simulink model "Glider_Sim_2015b"  (R2020a)
settings: Solver=ode45  StartTime=0.0  StopTime=10  MaxStep=0.1  RelTol=1e-3  EnableMultiTasking=on
InitFcn:
  | close all
  | AC=1; %Define Aircraft Case
  | SC_DynEqns; %Get the Stability Parameters
  | %[u alpha q theta beta p r phi]
  | XIC=[10. 6*pi/180. 0. 6*pi/180. 0*pi/180. 0. 0. 0*pi/180.]'; %Initial small perturbations
  | PsiIC=0.; %Initial Heading, radians
  | % clear the plot function to create new plots
  | % if you close the figure window, clear the function
  | % comment out the line below to overlay plots
  | clear PlotGlider
StartFcn:
  | tic
StopFcn:
  | toctime=toc;
  | xyz=xyz_E+[0 0 5000];
  | Score=0.3*(0.5*ceil(2*xyz(1))+4*abs(ceil(xyz(3))))+3*(abs(xyz(2))<=10);
  | fprintf('X-Dist = %5.1f    Score = %4.1f    Time= %3.1f sec\n',xyz(1),Score,tout(end))
  | str=(['X-Dist = ' num2str(xyz(1)) '    Score = ' num2str(Score)]);
values from neighbouring files (symbols this model uses):
  A = [Along zeros(4,4);zeros(4,4) Ald]    [SC_DynEqns.m]
  Alt = 5006    [AC_Data3.m]
  fps2kt = 0.5924838013    [AC_Data3.m]
  r2d = 180/pi    (= 57.2957795131)    [AC_Data3.m]
  tht = -0.086588    [AC_Data3.m]
  X0 = [U1 atrm 0 tht 0 0 0 0]'    [AC_Data3.m]
undefined symbols (not defined in the file or in its folder): PlotGlider
libraries: simulink x2
settings Model: Creator=bordignk  LastModifiedBy=Edward Han
settings DataIOCC: SaveFormat=Array  SignalLoggingSaveFormat=ModelDataLogs  ReturnWorkspaceOutputs=off
settings OptimizationCC: ExpressionDepthLimit=2147483647  InitFltsAndDblsToZero=on  LifeSpan=inf
settings DebuggingCC: UnderspecifiedInitializationDetection=Classic  MergeDetectMultiDrivingBlocksExec=none  FcnCallInpInsideContextMsg=warning  UnconnectedInputMsg=none  UnconnectedOutputMsg=none  AllowSymbolicDim=off  StateNameClashWarn=warning  SFUnexpectedBacktrackingDiag=warning  SFNoUnconditionalDefaultTransitionDiag=warning  SFExecutionAtInitializationDiag=none  ArithmeticOperatorsInVariantConditions=warning
settings HardwareCC: ProdBitPerPointer=32  ProdBitPerSizeT=32  ProdBitPerPtrDiffT=32  ProdLargestAtomicFloat=None  ProdIntDivRoundTo=Undefined  ProdEndianess=Unspecified  ProdWordSize=32  ProdHWDeviceType=32-bit Generic
settings ModelReferenceCC: PropagateSignalLabelsOutOfModel=off
settings SFSimCC: SimUseLocalCustomCode=off  SimParseCustomCode=off  CustomCodeUndefinedFunction=UseInterfaceOnly
settings RTWCC: RTWUseLocalCustomCode=off
settings CodeAppCC: StateflowObjectComments=on
settings GRTTargetCC: TargetLangStandard=C89/C90 (ANSI)  CombineOutputUpdateFcns=off  GRTInterface=on
settings ConfigComp: CovMetricSettings=dw  CovHtmlReporting=on  CovSaveCumulativeToWorkspaceVar=on  CovSaveSingleToWorkspaceVar=on  CovExternalEMLEnable=off  CovSFcnEnable=off

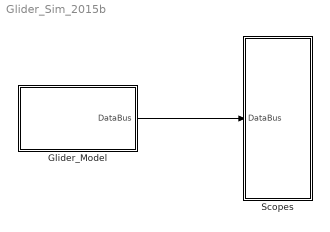
== system Glider_Sim_2015b ==
  Glider_Model : Subsystem
  Scopes : Subsystem
  wires:
  Glider_Model/1(DataBus) -> Scopes/1(DataBus)

== system Glider_Sim_2015b/Glider_Model ==
  Gain2 : Gain  Gain=A  Multiplication=Matrix(K*u)
  Integrator : Integrator  InitialCondition=XIC
  Make_Data : Subsystem
  DataBus : Outport  VectorParamsAs1DForOutWhenUnconnected=off
  wires:
  Gain2/1 -> Integrator/1, Make_Data/1(xdt)  "xdt"
  Make_Data/1(DataBus) -> DataBus/1
  Integrator/1 -> Make_Data/2(x)  "x"
  Make_Data/2(x_out) -> Gain2/1

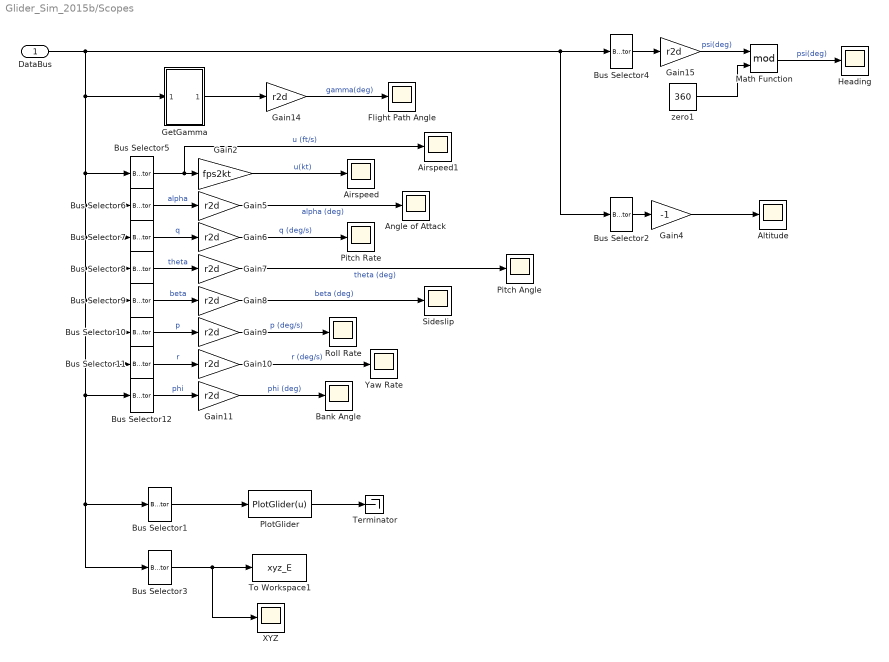
== system Glider_Sim_2015b/Scopes ==
  DataBus : Inport
  Airspeed : Scope
  Airspeed1 : Scope
  Altitude : Scope
  Angle of Attack : Scope
  Bank Angle : Scope
  Bus Selector1 : BusSelector  OutputSignals=Xe_ft,ye_ft,ze_ft,phi_rad,theta_rad,psi_rad  OutputAsBus=on
  Bus Selector10 : BusSelector  OutputSignals=p_rps  OutputAsBus=on
  Bus Selector11 : BusSelector  OutputSignals=r_rps  OutputAsBus=on
  Bus Selector12 : BusSelector  OutputSignals=phi_rad  OutputAsBus=on
  Bus Selector2 : BusSelector  OutputSignals=ze_ft  OutputAsBus=on
  Bus Selector3 : BusSelector  OutputSignals=Xe_ft,ye_ft,ze_ft  OutputAsBus=on
  Bus Selector4 : BusSelector  OutputSignals=psi_rad  OutputAsBus=on
  Bus Selector5 : BusSelector  OutputSignals=v_fps  OutputAsBus=on
  Bus Selector6 : BusSelector  OutputSignals=alpha_rad  OutputAsBus=on
  Bus Selector7 : BusSelector  OutputSignals=q_rps  OutputAsBus=on
  Bus Selector8 : BusSelector  OutputSignals=theta_rad  OutputAsBus=on
  Bus Selector9 : BusSelector  OutputSignals=beta_rad  OutputAsBus=on
  Flight Path Angle : Scope
  Gain{5..11,14..15} (9 alike) : Gain  Gain=r2d
  Gain2 : Gain  Gain=fps2kt
  Gain4 : Gain  Gain=-1
  GetGamma : Subsystem
  Heading : Scope
  Math Function : Math  Operator=mod  SignedPower=on  SaturateOnIntegerOverflow=on
  Pitch Angle : Scope
  Pitch Rate : Scope
  PlotGlider : MATLABFcn  MATLABFcn=PlotGlider(u)
  Roll Rate : Scope
  Sideslip : Scope
  Terminator : Terminator
  To Workspace1 : ToWorkspace  VariableName=xyz_E  SampleTime=-1
      settings: MaxDataPoints=1
  XYZ : Scope
  Yaw Rate : Scope
  zero1 : Constant  Value=360
  wires:
  DataBus/1 -> Bus Selector5/1, Bus Selector6/1, Bus Selector7/1, Bus Selector8/1, Bus Selector9/1, Bus Selector10/1, Bus Selector11/1, Bus Selector12/1, Bus Selector1/1, Bus Selector3/1, GetGamma/1(In1), Bus Selector4/1, Bus Selector2/1
  Math Function/1 -> Heading/1  "psi(deg)"
  Bus Selector2/1 -> Gain4/1
  Gain4/1 -> Altitude/1
  Bus Selector4/1 -> Gain15/1
  Bus Selector5/1 -> Airspeed1/1, Gain2/1  "u (ft/s)"
  Bus Selector6/1 -> Gain5/1  "alpha"
  Bus Selector7/1 -> Gain6/1  "q"
  Bus Selector8/1 -> Gain7/1  "theta"
  Bus Selector9/1 -> Gain8/1  "beta"
  Bus Selector10/1 -> Gain9/1  "p"
  Bus Selector11/1 -> Gain10/1  "r"
  Bus Selector12/1 -> Gain11/1  "phi"
  Gain5/1 -> Angle of Attack/1  "alpha (deg)"
  Gain6/1 -> Pitch Rate/1  "q (deg/s)"
  Gain7/1 -> Pitch Angle/1  "theta (deg)"
  Gain8/1 -> Sideslip/1  "beta (deg)"
  Gain9/1 -> Roll Rate/1  "p (deg/s)"
  Gain10/1 -> Yaw Rate/1  "r (deg/s)"
  Gain11/1 -> Bank Angle/1  "phi (deg)"
  Gain2/1 -> Airspeed/1  "u(kt)"
  Gain15/1 -> Math Function/1  "psi(deg)"
  zero1/1 -> Math Function/2
  Gain14/1 -> Flight Path Angle/1  "gamma(deg)"
  Bus Selector1/1 -> PlotGlider/1
  PlotGlider/1 -> Terminator/1
  GetGamma/1(Out1) -> Gain14/1
  Bus Selector3/1 -> XYZ/1, To Workspace1/1

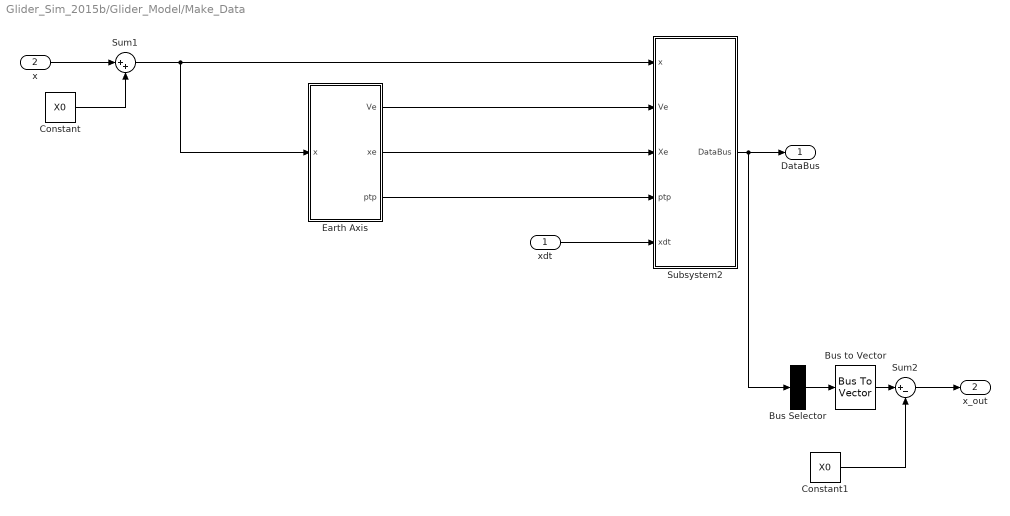
== system Glider_Sim_2015b/Glider_Model/Make_Data ==
  xdt : Inport  PortDimensions=[8 1]
  x : Inport  Port=2  PortDimensions=[8 1]
  Bus Selector : BusSelector  OutputSignals=v_fps,alpha_rad,q_rps,theta_rad,beta_rad,p_rps,r_rps,phi_rad  OutputAsBus=on
  Bus to Vector : BusToVector
  Constant : Constant  Value=X0
  Constant1 : Constant  Value=X0
  Earth Axis : Subsystem
  Subsystem2 : Subsystem
  Sum1 : Sum  Inputs=|++
  Sum2 : Sum  Inputs=|+-
  DataBus : Outport  VectorParamsAs1DForOutWhenUnconnected=off
  x_out : Outport  Port=2  VectorParamsAs1DForOutWhenUnconnected=off
  wires:
  x/1 -> Sum1/1
  Constant/1 -> Sum1/2
  Sum1/1 -> Subsystem2/1(x), Earth Axis/1(x)
  Earth Axis/2(xe) -> Subsystem2/3(Xe)
  xdt/1 -> Subsystem2/5(xdt)
  Subsystem2/1(DataBus) -> Bus Selector/1, DataBus/1
  Earth Axis/1(Ve) -> Subsystem2/2(Ve)
  Earth Axis/3(ptp) -> Subsystem2/4(ptp)
  Bus Selector/1 -> Bus to Vector/1
  Bus to Vector/1 -> Sum2/1
  Constant1/1 -> Sum2/2
  Sum2/1 -> x_out/1

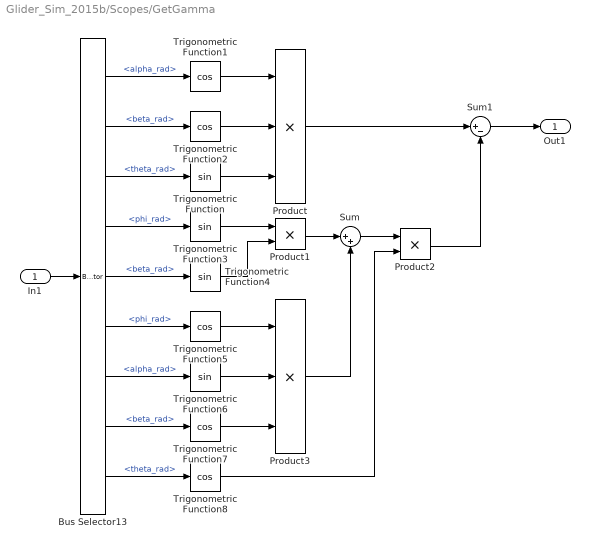
== system Glider_Sim_2015b/Scopes/GetGamma ==
  In1 : Inport
  Bus Selector13 : BusSelector  OutputSignals=alpha_rad,beta_rad,theta_rad,phi_rad,beta_rad,phi_rad,alpha_rad,beta_rad,theta_rad
  Product : Product  Inputs=3
  Product1 : Product
  Product2 : Product
  Product3 : Product  Inputs=3
  Sum : Sum  Inputs=|++
  Sum1 : Sum  Inputs=|+-
  Trigonometric Function{,3..4,6} (4 alike) : Trigonometry
  Trigonometric Function{1..2,5,7..8} (5 alike) : Trigonometry  Operator=cos
  Out1 : Outport  VectorParamsAs1DForOutWhenUnconnected=off
  wires:
  Sum1/1 -> Out1/1
  In1/1 -> Bus Selector13/1
  Bus Selector13/1 -> Trigonometric Function1/1  "<alpha_rad>"
  Bus Selector13/2 -> Trigonometric Function2/1  "<beta_rad>"
  Bus Selector13/3 -> Trigonometric Function/1  "<theta_rad>"
  Bus Selector13/4 -> Trigonometric Function3/1  "<phi_rad>"
  Bus Selector13/5 -> Trigonometric Function4/1  "<beta_rad>"
  Bus Selector13/6 -> Trigonometric Function5/1  "<phi_rad>"
  Bus Selector13/7 -> Trigonometric Function6/1  "<alpha_rad>"
  Bus Selector13/8 -> Trigonometric Function7/1  "<beta_rad>"
  Bus Selector13/9 -> Trigonometric Function8/1  "<theta_rad>"
  Trigonometric Function1/1 -> Product/1
  Trigonometric Function2/1 -> Product/2
  Trigonometric Function/1 -> Product/3
  Product/1 -> Sum1/1
  Trigonometric Function3/1 -> Product1/1
  Trigonometric Function4/1 -> Product1/2
  Trigonometric Function5/1 -> Product3/1
  Trigonometric Function6/1 -> Product3/2
  Trigonometric Function7/1 -> Product3/3
  Product1/1 -> Sum/1
  Product3/1 -> Sum/2
  Sum/1 -> Product2/1
  Trigonometric Function8/1 -> Product2/2
  Product2/1 -> Sum1/2

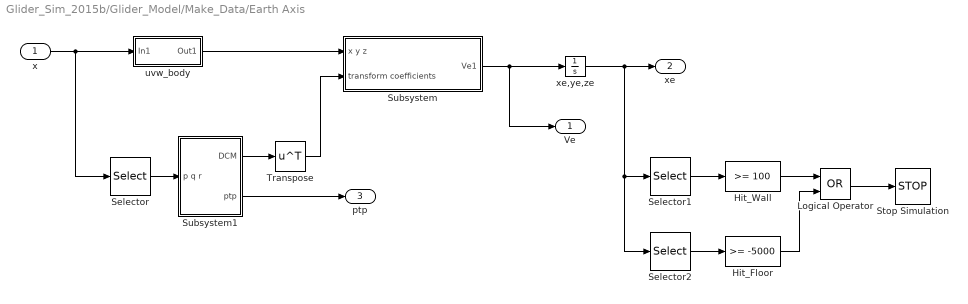
== system Glider_Sim_2015b/Glider_Model/Make_Data/Earth Axis ==
  x : Inport
  Hit_Floor : simulink/Logic and Bit Operations/Compare To Constant  relop=>=  const=-5000  OutDataTypeStr=boolean
  Hit_Wall : simulink/Logic and Bit Operations/Compare To Constant  relop=>=  const=100  OutDataTypeStr=boolean
  Logical Operator : Logic  Operator=OR  AllPortsSameDT=off  OutDataTypeStr=boolean
  Selector : Selector  InputPortWidth=8  IndexOptions=Index vector (dialog)  Indices=[6 3 7]  OutputSizes=1
  Selector1 : Selector  InputPortWidth=3  IndexOptions=Index vector (dialog)  Indices=[1]  OutputSizes=1
  Selector2 : Selector  InputPortWidth=3  IndexOptions=Index vector (dialog)  Indices=[3]  OutputSizes=1
  Stop Simulation : Stop
  Subsystem : Subsystem
  Subsystem1 : Subsystem
  Transpose : Math  Operator=transpose  SignedPower=on  SaturateOnIntegerOverflow=on
  uvw_body : Subsystem
  xe,ye,ze : Integrator  InitialCondition=[0 0 -Alt]
  Ve : Outport  VectorParamsAs1DForOutWhenUnconnected=off
  xe : Outport  Port=2  VectorParamsAs1DForOutWhenUnconnected=off
  ptp : Outport  Port=3  VectorParamsAs1DForOutWhenUnconnected=off
  wires:
  Subsystem1/1(DCM) -> Transpose/1
  Transpose/1 -> Subsystem/2(transform coefficients)
  Selector/1 -> Subsystem1/1("p q r ")
  uvw_body/1(Out1) -> Subsystem/1(x y z)
  x/1 -> Selector/1, uvw_body/1(In1)
  xe,ye,ze/1 -> Selector2/1, Selector1/1, xe/1
  Subsystem/1(Ve1) -> xe,ye,ze/1, Ve/1
  Selector1/1 -> Hit_Wall/1
  Selector2/1 -> Hit_Floor/1
  Hit_Wall/1 -> Logical Operator/1
  Hit_Floor/1 -> Logical Operator/2
  Logical Operator/1 -> Stop Simulation/1
  Subsystem1/2(ptp) -> ptp/1

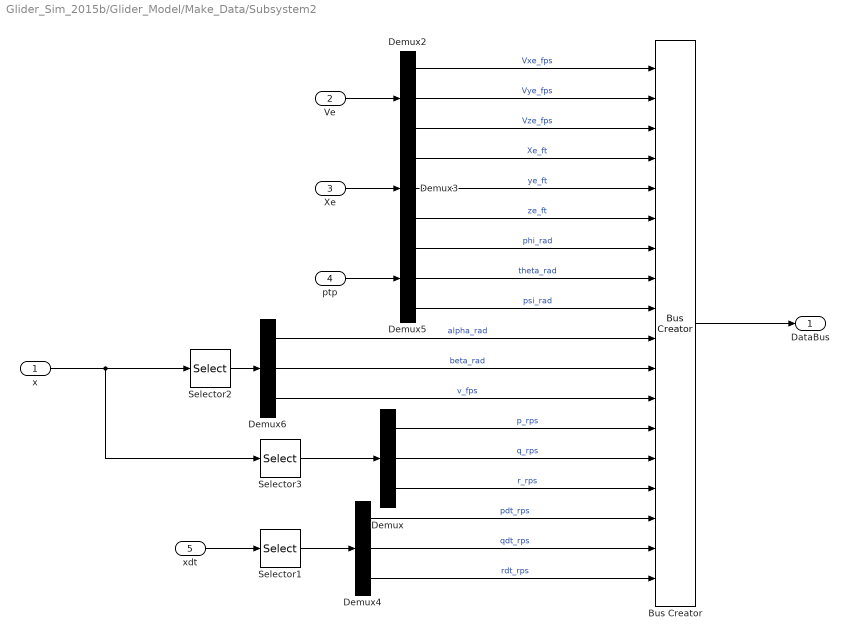
== system Glider_Sim_2015b/Glider_Model/Make_Data/Subsystem2 ==
  x : Inport
  Ve : Inport  Port=2
  Xe : Inport  Port=3
  ptp : Inport  Port=4
  xdt : Inport  Port=5
  Bus Creator : BusCreator  Inputs=18
  Demux{,2..6} (6 alike) : Demux  Outputs=3
  Selector1 : Selector  InputPortWidth=8  IndexOptions=Index vector (dialog)  Indices=[6 3 7]  OutputSizes=1
  Selector2 : Selector  InputPortWidth=8  IndexOptions=Index vector (dialog)  Indices=[2 5 1]  OutputSizes=1
  Selector3 : Selector  InputPortWidth=8  IndexOptions=Index vector (dialog)  Indices=[6 3 7]  OutputSizes=1
  DataBus : Outport  VectorParamsAs1DForOutWhenUnconnected=off
  wires:
  Selector2/1 -> Demux6/1
  x/1 -> Selector3/1, Selector2/1
  Demux4/3 -> Bus Creator/18  "rdt_rps"
  Demux4/2 -> Bus Creator/17  "qdt_rps"
  Demux4/1 -> Bus Creator/16  "pdt_rps"
  Demux/3 -> Bus Creator/15  "r_rps"
  Demux/2 -> Bus Creator/14  "q_rps"
  Demux/1 -> Bus Creator/13  "p_rps"
  Demux6/3 -> Bus Creator/12  "v_fps"
  Demux6/2 -> Bus Creator/11  "beta_rad"
  Demux6/1 -> Bus Creator/10  "alpha_rad"
  Demux5/3 -> Bus Creator/9  "psi_rad"
  Demux5/2 -> Bus Creator/8  "theta_rad"
  Demux5/1 -> Bus Creator/7  "phi_rad"
  Demux3/3 -> Bus Creator/6  "ze_ft"
  Demux3/2 -> Bus Creator/5  "ye_ft"
  Demux3/1 -> Bus Creator/4  "Xe_ft"
  Demux2/3 -> Bus Creator/3  "Vze_fps"
  Demux2/2 -> Bus Creator/2  "Vye_fps"
  Demux2/1 -> Bus Creator/1  "Vxe_fps"
  xdt/1 -> Selector1/1
  Xe/1 -> Demux3/1
  Ve/1 -> Demux2/1
  Selector3/1 -> Demux/1
  Selector1/1 -> Demux4/1
  ptp/1 -> Demux5/1
  Bus Creator/1 -> DataBus/1

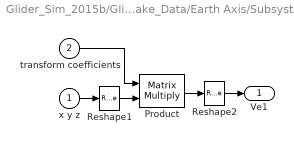
== system Glider_Sim_2015b/Glider_Model/Make_Data/Earth Axis/Subsystem ==
  x y z : Inport
  transform coefficients : Inport  Port=2
  Product : Product  Multiplication=Matrix(*)  InputSameDT=on  SaturateOnIntegerOverflow=on  OutDataTypeStr=Inherit: Same as first input
  Reshape1 : Reshape  OutputDimensionality=Column vector (2-D)
  Reshape2 : Reshape
  Ve1 : Outport  VectorParamsAs1DForOutWhenUnconnected=off
  wires:
  Reshape2/1 -> Ve1/1
  Reshape1/1 -> Product/2
  x y z/1 -> Reshape1/1
  transform coefficients/1 -> Product/1
  Product/1 -> Reshape2/1

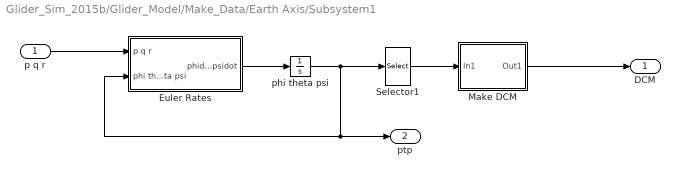
== system Glider_Sim_2015b/Glider_Model/Make_Data/Earth Axis/Subsystem1 ==
  "p q r " : Inport
  Euler Rates : Subsystem
  Make DCM : Subsystem
  Selector1 : Selector  InputPortWidth=3  IndexOptions=Index vector (dialog)  Indices=[3 2 1]  OutputSizes=1
  phi theta psi : Integrator  InitialCondition=[0 tht 0]+([XIC([8 4])' PsiIC])
  DCM : Outport  VectorParamsAs1DForOutWhenUnconnected=off
  ptp : Outport  Port=2  VectorParamsAs1DForOutWhenUnconnected=off
  wires:
  Selector1/1 -> Make DCM/1(In1)
  phi theta psi/1 -> Selector1/1, ptp/1, Euler Rates/2(phi theta psi)
  Euler Rates/1(phidot thetadot psidot) -> phi theta psi/1
  "p q r "/1 -> Euler Rates/1(p q r)
  Make DCM/1(Out1) -> DCM/1

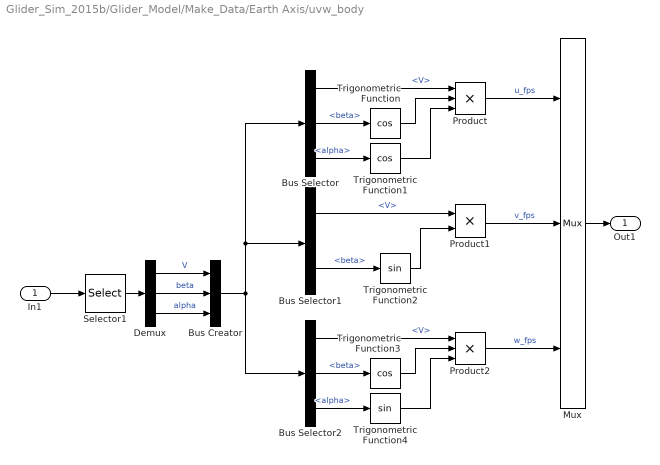
== system Glider_Sim_2015b/Glider_Model/Make_Data/Earth Axis/uvw_body ==
  In1 : Inport
  Bus Creator : BusCreator  Inputs=3
  Bus Selector : BusSelector  OutputSignals=V,beta,alpha
  Bus Selector1 : BusSelector  OutputSignals=V,beta
  Bus Selector2 : BusSelector  OutputSignals=V,beta,alpha
  Demux : Demux  Outputs=3
  Mux : Mux  Inputs=3
  Product : Product  Inputs=3  RndMeth=Zero
  Product1 : Product  RndMeth=Zero
  Product2 : Product  Inputs=3  RndMeth=Zero
  Selector1 : Selector  InputPortWidth=8  IndexOptions=Index vector (dialog)  Indices=[1 5 2]  OutputSizes=1
  Trigonometric Function : Trigonometry  Operator=cos
  Trigonometric Function1 : Trigonometry  Operator=cos
  Trigonometric Function2 : Trigonometry
  Trigonometric Function3 : Trigonometry  Operator=cos
  Trigonometric Function4 : Trigonometry
  Out1 : Outport  VectorParamsAs1DForOutWhenUnconnected=off
  wires:
  Selector1/1 -> Demux/1
  Demux/1 -> Bus Creator/1  "V"
  Demux/2 -> Bus Creator/2  "beta"
  Demux/3 -> Bus Creator/3  "alpha"
  Bus Creator/1 -> Bus Selector/1, Bus Selector1/1, Bus Selector2/1
  Bus Selector/2 -> Trigonometric Function/1  "<beta>"
  Bus Selector/3 -> Trigonometric Function1/1  "<alpha>"
  Bus Selector/1 -> Product/1  "<V>"
  Trigonometric Function/1 -> Product/2
  Trigonometric Function1/1 -> Product/3
  Bus Selector1/2 -> Trigonometric Function2/1  "<beta>"
  Bus Selector1/1 -> Product1/1  "<V>"
  Trigonometric Function2/1 -> Product1/2
  Bus Selector2/2 -> Trigonometric Function3/1  "<beta>"
  Bus Selector2/3 -> Trigonometric Function4/1  "<alpha>"
  Bus Selector2/1 -> Product2/1  "<V>"
  Trigonometric Function3/1 -> Product2/2
  Trigonometric Function4/1 -> Product2/3
  Product/1 -> Mux/1  "u_fps"
  Product1/1 -> Mux/2  "v_fps"
  Product2/1 -> Mux/3  "w_fps"
  In1/1 -> Selector1/1
  Mux/1 -> Out1/1

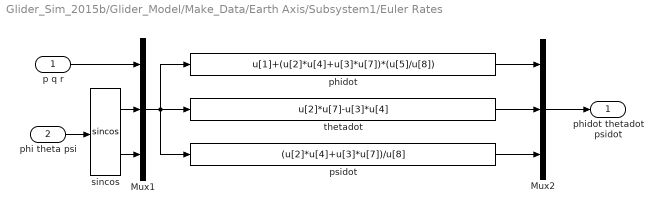
== system Glider_Sim_2015b/Glider_Model/Make_Data/Earth Axis/Subsystem1/Euler Rates ==
  p q r : Inport
  phi theta psi : Inport  Port=2
  Mux1 : Mux  Inputs=[3 3 3]
  Mux2 : Mux  Inputs=3
  phidot : Fcn  Expr=u[1]+(u[2]*u[4]+u[3]*u[7])*(u[5]/u[8])
  psidot : Fcn  Expr=(u[2]*u[4]+u[3]*u[7])/u[8]
  sincos : Trigonometry  Operator=sincos
  thetadot : Fcn  Expr=u[2]*u[7]-u[3]*u[4]
  phidot thetadot psidot : Outport  InitialOutput=0  VectorParamsAs1DForOutWhenUnconnected=off
  wires:
  Mux1/1 -> psidot/1, phidot/1, thetadot/1
  p q r/1 -> Mux1/1
  phi theta psi/1 -> sincos/1
  psidot/1 -> Mux2/3
  thetadot/1 -> Mux2/2
  phidot/1 -> Mux2/1
  Mux2/1 -> phidot thetadot psidot/1
  sincos/1 -> Mux1/2
  sincos/2 -> Mux1/3

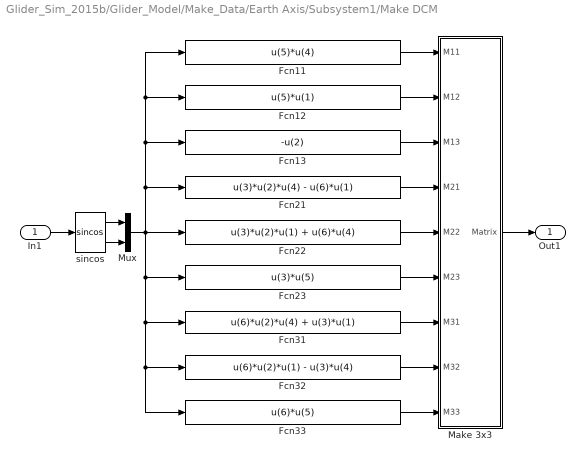
== system Glider_Sim_2015b/Glider_Model/Make_Data/Earth Axis/Subsystem1/Make DCM ==
  In1 : Inport  PortDimensions=3
  Fcn11 : Fcn  Expr=u(5)*u(4)
  Fcn12 : Fcn  Expr=u(5)*u(1)
  Fcn13 : Fcn  Expr=-u(2)
  Fcn21 : Fcn  Expr=u(3)*u(2)*u(4) - u(6)*u(1)
  Fcn22 : Fcn  Expr=u(3)*u(2)*u(1) + u(6)*u(4)
  Fcn23 : Fcn  Expr=u(3)*u(5)
  Fcn31 : Fcn  Expr=u(6)*u(2)*u(4) + u(3)*u(1)
  Fcn32 : Fcn  Expr=u(6)*u(2)*u(1) - u(3)*u(4)
  Fcn33 : Fcn  Expr=u(6)*u(5)
  Make 3x3 : Subsystem
  Mux : Mux  Inputs=2
  sincos : Trigonometry  Operator=sincos
  Out1 : Outport  PortDimensions=[3,3]  VectorParamsAs1DForOutWhenUnconnected=off
  wires:
  In1/1 -> sincos/1
  Make 3x3/1(Matrix) -> Out1/1
  sincos/1 -> Mux/1
  sincos/2 -> Mux/2
  Mux/1 -> Fcn32/1, Fcn33/1, Fcn31/1, Fcn23/1, Fcn22/1, Fcn11/1, Fcn12/1, Fcn13/1, Fcn21/1
  Fcn11/1 -> Make 3x3/1(M11)
  Fcn12/1 -> Make 3x3/2(M12)
  Fcn13/1 -> Make 3x3/3(M13)
  Fcn21/1 -> Make 3x3/4(M21)
  Fcn22/1 -> Make 3x3/5(M22)
  Fcn23/1 -> Make 3x3/6(M23)
  Fcn31/1 -> Make 3x3/7(M31)
  Fcn32/1 -> Make 3x3/8(M32)
  Fcn33/1 -> Make 3x3/9(M33)

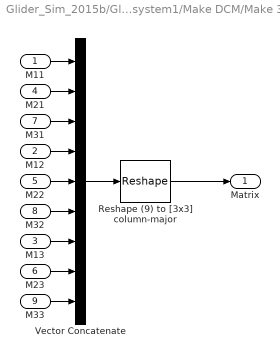
== system Glider_Sim_2015b/Glider_Model/Make_Data/Earth Axis/Subsystem1/Make DCM/Make 3x3 ==
  M11 : Inport  PortDimensions=1
  M12 : Inport  Port=2  PortDimensions=1
  M13 : Inport  Port=3  PortDimensions=1
  M21 : Inport  Port=4  PortDimensions=1
  M22 : Inport  Port=5  PortDimensions=1
  M23 : Inport  Port=6  PortDimensions=1
  M31 : Inport  Port=7  PortDimensions=1
  M32 : Inport  Port=8  PortDimensions=1
  M33 : Inport  Port=9  PortDimensions=1
  Reshape (9) to [3x3] column-major : Reshape  OutputDimensionality=Customize  OutputDimensions=[3,3]
  Vector Concatenate : Concatenate  NumInputs=9
  Matrix : Outport  PortDimensions=[3 3]  VectorParamsAs1DForOutWhenUnconnected=off
  wires:
  M33/1 -> Vector Concatenate/9
  M23/1 -> Vector Concatenate/8
  M13/1 -> Vector Concatenate/7
  M32/1 -> Vector Concatenate/6
  Reshape (9) to [3x3] column-major/1 -> Matrix/1
  M22/1 -> Vector Concatenate/5
  M12/1 -> Vector Concatenate/4
  M31/1 -> Vector Concatenate/3
  M21/1 -> Vector Concatenate/2
  M11/1 -> Vector Concatenate/1
  Vector Concatenate/1 -> Reshape (9) to [3x3] column-major/1
